simulink model "LLC_bidirectional"  (R2020b)
settings: Solver=ode23tb  StartTime=0.0  StopTime=3.0e-3  RelTol=1e-4  EnableMultiTasking=on
PreLoadFcn:
  | Fs=13000;    % Switching frequency (Hz)
  | Vf=0.6;        % Diode forward voltage (V)
  | Rs_fet=1e5;  % FET snubber resistance (ohms)
  | Cs_fet=1e-5;  % FET snubber capacitance (ohms)
libraries: powerlib x29, powerlib_meascontrol x3, pid_lib x1
Description:
  | Copyright 2008-2019 The MathWorks, Inc.
settings Model: Creator=MathWorks  LastModifiedBy=lauramarks2
settings SolverCC: SolverResetMethod=Robust
settings DataIOCC: SaveOutput=off  SignalLogging=off  DSMLogging=off  SaveTime=off  ReturnWorkspaceOutputs=off
settings OptimizationCC: LifeSpan=inf
settings DebuggingCC: ReadBeforeWriteMsg=DisableAll  WriteAfterWriteMsg=DisableAll  WriteAfterReadMsg=DisableAll  MultiTaskDSMMsg=none  UnconnectedLineMsg=none  SFUnexpectedBacktrackingDiag=warning  SFNoUnconditionalDefaultTransitionDiag=warning  SFExecutionAtInitializationDiag=none  ArithmeticOperatorsInVariantConditions=warning
settings ModelReferenceCC: UpdateModelReferenceTargets=IfOutOfDate
settings SFSimCC: SFSimEcho=off  SimUseLocalCustomCode=off  CustomCodeUndefinedFunction=UseInterfaceOnly
settings RTWCC: RTWUseLocalCustomCode=off
settings CodeAppCC: StateflowObjectComments=on
settings GRTTargetCC: TargetLangStandard=C89/C90 (ANSI)
settings ConfigComp: CovMetricSettings=dw  CovSaveCumulativeToWorkspaceVar=on  CovSaveSingleToWorkspaceVar=on  CovExternalEMLEnable=off
settings SimscapeCC: SimscapeNormalizeSystem=off  SimscapeNominalValues={1, 'bar'; 1, 'cm^3/s'; 1, 'bar*kg/s'; 1, 'kJ/kg'; 1, 'kW'; }

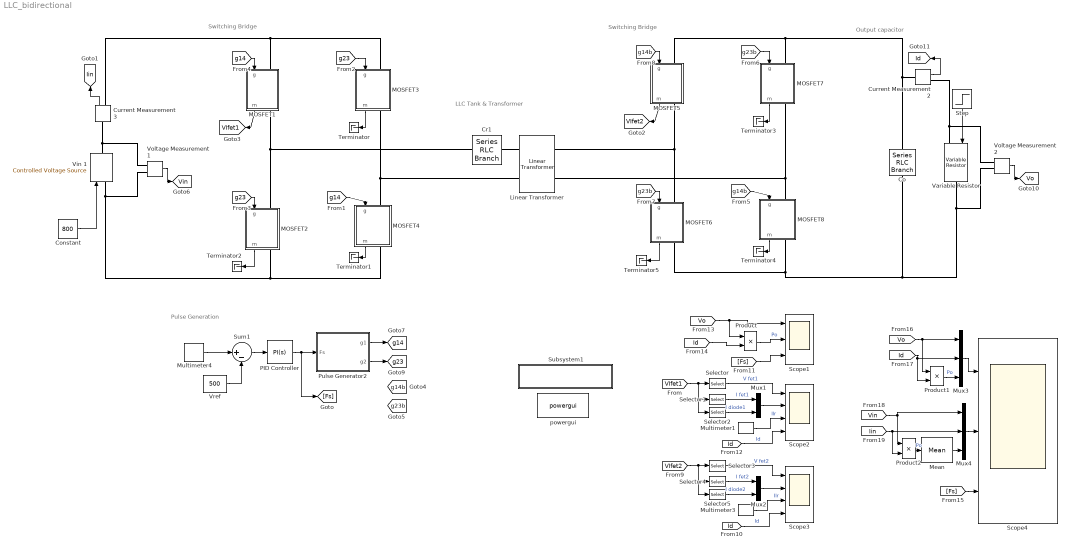
== system LLC_bidirectional ==
  note: Pulse Generation
  note: Switching Bridge
  note: Output capacitor
  note: LLC Tank & Transformer
  note: Switching Bridge
  Co : powerlib/Elements/Series RLC Branch  LConnTagsString=__new0  RConnTagsString=__new0  BranchType=C  Resistance=1e-4  Inductance=200e-6  SetiL0=off  InitialCurrent=0  Capacitance=100e-6  Setx0=on  InitialVoltage=0  Measurements=Branch voltage
  Constant : Constant  Value=800  OutDataTypeStr=double
  Cr1 : powerlib/Elements/Series RLC Branch  LConnTagsString=__new0  RConnTagsString=__new0  BranchType=C  Resistance=1e-4  Inductance=200e-6  SetiL0=off  InitialCurrent=0  Capacitance=1.5e-6  Setx0=off  InitialVoltage=40  Measurements=Branch voltage and current
  Current Measurement2 : powerlib/Measurements/Current Measurement  PhasorSimulation=off  OutputType=Complex  PSBequivalent=0
  Current Measurement3 : powerlib/Measurements/Current Measurement  PhasorSimulation=off  OutputType=Complex  PSBequivalent=0
  Linear Transformer : powerlib/Elements/Linear Transformer  UNITS=SI  NominalPower=[ 100e3 85e3 ]  winding1="[8   1e-2  2.02e-6]"  winding2="[5.7  1e-2  1.16e-6 ]"  ThreeWindings=off  winding3=[3.15e+05 0.7938 0.084225]  RmLm=[1e4 963e-6]  Measurements=All voltages and currents  DataType=on
  MOSFET1 : Subsystem
  MOSFET2 : Subsystem
  MOSFET3 : Subsystem
  MOSFET4 : Subsystem
  MOSFET5 : Subsystem
  MOSFET6 : Subsystem
  MOSFET7 : Subsystem
  MOSFET8 : Subsystem
  Mean : powerlib_meascontrol/Measurements/Mean  Freq=180e3  Vinit=0  Ts=0
  Multimeter1 : powerlib/Measurements/Multimeter  PhasorSimulation=off  OutputType=Complex  sel=1  L=10  Gain=0  yselected={}  PSBOutputType=1  PSBequivalent=0  AxesSetting=[0,0.1,-100,100]  Display=0  SavedBlockNames=-11
  Multimeter3 : powerlib/Measurements/Multimeter  PhasorSimulation=off  OutputType=Complex  sel=1  L=10  Gain=0  yselected={}  PSBOutputType=1  PSBequivalent=0  AxesSetting=[0,0.1,-100,100]  Display=0  SavedBlockNames=-11
  Multimeter4 : powerlib/Measurements/Multimeter  PhasorSimulation=off  OutputType=Complex  sel=1  L=10  Gain=1  yselected={'Ub: Co'};  PSBOutputType=1  PSBequivalent=0  AxesSetting=[0,0.1,-100,100]  Display=0  SavedBlockNames=-11
  Mux1 : Mux  Inputs=2
  Mux2 : Mux  Inputs=2
  Mux3 : Mux  Inputs=3
  Mux4 : Mux  Inputs=3
  PID Controller : pid_lib/PID Controller  Controller=PI  Form=Parallel  TimeDomain=Continuous-time  UseExternalTs=off  SampleTime=-1  IntegratorMethod=Forward Euler  FilterMethod=Forward Euler  ControllerParametersSource=internal  P=1200  I=1e-3  D=0  UseFilter=on  N=100  TunerSelectOption=Transfer Function Based (PID Tuner App)  InitialConditionSource=internal  InitialConditionForIntegrator=89e3  InitialConditionForFilter=0  DifferentiatorICPrevScaledInput=0  ExternalReset=none  TrackingMode=off  Kt=1  LimitOutput=off  SatLimitsSource=internal  UpperSaturationLimit=inf  LowerSaturationLimit=50e3  LinearizeAsGain=off  AntiWindupMode=none  Kb=1  POutMin=[]  POutMax=[]  IOutMin=[]  IOutMax=[]  DOutMin=[]  DOutMax=[]  NOutMin=[]  NOutMax=[]  SumOutMin=[]  SumOutMax=[]  SaturationOutMin=[]  SaturationOutMax=[]  PParamMin=[]  PParamMax=[]  IParamMin=[]  IParamMax=[]  DParamMin=[]  DParamMax=[]  NParamMin=[]  NParamMax=[]  KbParamMin=[]  KbParamMax=[]  KtParamMin=[]  KtParamMax=[]  KbOutMin=[]  KbOutMax=[]  KtOutMin=[]  KtOutMax=[]  IntegratorOutMin=[]  IntegratorOutMax=[]  FilterOutMin=[]  FilterOutMax=[]  SumI1OutMin=[]  SumI1OutMax=[]  SumI2OutMin=[]  SumI2OutMax=[]  SumI3OutMin=[]  SumI3OutMax=[]  SumI4OutMin=[]  SumI4OutMax=[]  SumDOutMin=[]  SumDOutMax=[]  DifferentiatorOutMin=[]  DifferentiatorOutMax=[]  FilterDiffOutCoefMin=[]  FilterDiffOutCoefMax=[]  ReciprocalOutMin=[]  ReciprocalOutMax=[]  SumDenOutMin=[]  SumDenOutMax=[]  SumNumOutMin=[]  SumNumOutMax=[]  DivideOutMin=[]  DivideOutMax=[]  UdiffTsProdOutMin=[]  UdiffTsProdOutMax=[]  NTsProdOutMin=[]  NTsProdOutMax=[]  UintegralTsProdOutMin=[]  UintegralTsProdOutMax=[]  UngainTsProdOutMin=[]  UngainTsProdOutMax=[]  IntegratorContinuousStateAttributes=''  IntegratorStateMustResolveToSignalObject=off  IntegratorRTWStateStorageClass=Auto  FilterContinuousStateAttributes=''  FilterStateMustResolveToSignalObject=off  FilterRTWStateStorageClass=Auto  ParallelPVariant=InternalParameters  IdealPVariant=Disabled  IVariant=InternalParameters  DVariant=Disabled  IntegratorVariant=Continuous  SatVariant=Disabled  AWVariant=Passthrough  PCopyVariant=Disabled  TRVariant=Disabled  FdbkBlocksVariant=Forward  IdealPFdbkVariant=Disabled  SatFdbkVariant=Disabled  DerivativeFilterVariant=Disabled  NVariant=Disabled  NCopyVariant=Disabled_SignalSpec  FilterICVariant=Disabled  IntegratorICVariant=InternalICs  ExternalResetVariant=Disabled  TRSumVariant=Passthrough  SumFdbkVariant=Disabled  SumVariant=Sum_PI  TsampFilterVariant=InternalTs  TsampNgainVariant=Passthrough  TsampIntegralVariant=Passthrough  ExternalSaturationOutDataTypeStr=Inherit: Same as second input
  Product : Product
  Product1 : Product
  Product2 : Product
  Pulse Generator2 : Subsystem
  "Scope1 " : Scope  NumInputPorts=3
  Scope2 : Scope  NumInputPorts=4
  Scope3 : Scope  NumInputPorts=4
  Scope4 : Scope  NumInputPorts=3
  Selector : Selector  InputPortWidth=3  IndexOptions=Index vector (dialog)  Indices=2  OutputSizes=1
  Selector1 : Selector  InputPortWidth=3  IndexOptions=Index vector (dialog)  Indices=1  OutputSizes=1
  Selector2 : Selector  InputPortWidth=3  IndexOptions=Index vector (dialog)  Indices=3  OutputSizes=1
  Selector3 : Selector  InputPortWidth=3  IndexOptions=Index vector (dialog)  Indices=2  OutputSizes=1
  Selector4 : Selector  InputPortWidth=3  IndexOptions=Index vector (dialog)  Indices=1  OutputSizes=1
  Selector5 : Selector  InputPortWidth=3  IndexOptions=Index vector (dialog)  Indices=3  OutputSizes=1
  Step : Step  Time=2e-3  Before=2.5  After=2.5  SampleTime=1e-5
  Subsystem1 : Subsystem
      settings: OpenFcn=|
      | %
      | L=10e-6;
      | C=20e-6;
      | Freq=[1000:1:50000];
      | w=2*pi*Freq;
      | Fo=1/(2*pi*sqrt(L*C));
      | wo=2*pi*Fo;
      | %
      | Rload=[0.5 5];
      | R=8/(pi^2)*Rload;
      | %
      | for n=1:2
      | Q(n)=sqrt(L/C)/R(n);
      |     Zeta(n)=1/(2*Q(n));
      |     s=j*w;
      |     Num(n,:)= (2*Zeta(n)*wo).*s;
      |     Den(n,:)= s.^2 + (2*Zeta(n)*wo).*s + wo^2;
      |     K(n,:)=Num(n,:)./Den(n,:);
      | end
      | figure(1)
      | clf
      | ScreenS=get(0,'Screensize');
      | x0=ScreenS(3); y0=ScreenS(4);
      | PositionParam=[x0/4 y0/8 x0/2 y0/1.4];
      | set(gcf,'Position',PositionParam);
      | subplot(2,1,1)
      | plot(Freq/1000, abs(K(1,:)),'b')
      | hold on
      | plot(Freq/1000, abs(K(2,:)),'r')
      | xlabel('Fs (kHz)')
      | grid
      | axis([0 40 0 1.1])
      | legend('Rload=0.5 ohms', 'Rload=5 ohms','Location', 'NorthEast')
      | title('DC Gain Characteristic - Magnitude')
      | %
      | subplot(2,1,2)
      | plot(Freq/1000, angle(K(1,:))*180/pi,'b')
      | hold on
      | plot(Freq/1000, angle(K(2,:))*180/pi,'r')
      | xlabel('Fs (kHz)')
      | ylabel('Degrees')
      | grid
      | axis([0 40 -100 100])
      | legend('Rload=0.5 ohms', 'Rload=5 ohms','Location', 'NorthEast')
      | title('DC Gain Characteristic - Phase')
      mask Display: disp('Plot Theoretical\nDC Gain Characteristic')
  Sum1 : Sum  Inputs=|+-  InputSameDT=on  SaturateOnIntegerOverflow=on  OutDataTypeStr=Inherit: Same as first input
  Terminator{,1..5} (6 alike) : Terminator
  Variable Resistor : powerlib/Elements/Variable Resistor  Rabsmin=1e-3
      settings: SourceProductBaseCode=PS
  Vin 1 : powerlib/Electrical Sources/Controlled Voltage Source  Initialize=on  Source_Type=AC  Amplitude=0  Phase=0  Frequency=0  Measurements=None
  Voltage Measurement1 : powerlib/Measurements/Voltage Measurement  PhasorSimulation=off  OutputType=Complex  PSBequivalent=0
  Voltage Measurement2 : powerlib/Measurements/Voltage Measurement  PhasorSimulation=off  OutputType=Complex  PSBequivalent=0
  Vref : Constant  Value=500
  powergui : powerlib/powergui  Priority=1  SimulationMode=Discrete  SampleTime=1e-8  frequency=60  Iterations=50  frequencyindice=0  Pbase=100e6  ErrMax=1e-4  UnitsV=kV  UnitsW=MW  buscounter=0  FunctionMessages=off  echomessages=off  EnableUseOfTLC=off  CurrentSourceSwitches=off  DisableSnubberDevices=off  DisableRonSwitches=off  DisableVfSwitches=off  DisplayEquations=off  AutomaticDiscreteSolvers=off  SolverType=Tustin/Backward Euler (TBE)  Interpol=off  ExternalGateDelay=off  methode=off  Ts=100  x0status=blocks  SPID=on  SwTol=0  HookPort=off  NonlinearTolerance=0  nMaxIteration=15  ContinueOnMaxIteration=off  RestoreLinks=warning  ResistiveCurrentMeasurement=off  Frange=[1000:0.5:40000]  Ylog=off  Xlog=off  ShowGrid=off  save=off  variable=ZData  structure=0  ZoomFFT=off  StartTime=0.0  cycles=1  DisplayStyle=1  fundamental=60  FreqAxis=off  MaxFrequency=1000  frequencyindicesteady=1  RmsSteady=1  display=off
  tag scope: Id=global, Iin=global, VIfet1=global, VIfet2=global, Vin=global, Vo=global, g14=global, g14b=global, g23=global, g23b=global
  wires:
  [g23] -> MOSFET2/1(g)
  [g14] -> MOSFET1/1(g)
  MOSFET1/1(m) -> [VIfet1]
  Product/1 -> "Scope1 "/2  "Po"
  [g14] -> MOSFET4/1(g)
  [g23] -> MOSFET3/1(g)
  Mux1/1 -> Scope2/2
  Selector2/1 -> Mux1/2  "I diode1"
  [Id] -> Scope2/4  "Id"
  Multimeter1/1 -> Scope2/3  "Ilr"
  Selector1/1 -> Mux1/1  "I fet1"
  MOSFET3/1(m) -> Terminator/1
  MOSFET4/1(m) -> Terminator1/1
  MOSFET2/1(m) -> Terminator2/1
  [VIfet1] -> Selector2/1, Selector1/1, Selector/1
  Selector/1 -> Scope2/1  "V fet1"
  Current Measurement3/1 -> [Iin]
  Voltage Measurement1/1 -> [Vin]
  MOSFET7/1(m) -> Terminator3/1
  [g23b] -> MOSFET6/1(g)
  [g14b] -> MOSFET8/1(g)
  [g23b] -> MOSFET7/1(g)
  MOSFET5/1(m) -> [VIfet2]
  MOSFET6/1(m) -> Terminator5/1
  [g14b] -> MOSFET5/1(g)
  MOSFET8/1(m) -> Terminator4/1
  Multimeter3/1 -> Scope3/3  "Ilr"
  [Id] -> Scope3/4  "Id"
  Mux2/1 -> Scope3/2
  Selector4/1 -> Mux2/1  "I fet2"
  Selector3/1 -> Scope3/1  "V fet2"
  [VIfet2] -> Selector5/1, Selector4/1, Selector3/1
  Selector5/1 -> Mux2/2  "I diode2"
  Multimeter4/1 -> Sum1/1
  Sum1/1 -> PID Controller/1
  Vref/1 -> Sum1/2
  Pulse Generator2/2(g2) -> [g23]
  Pulse Generator2/1(g1) -> [g14]
  [Fs] -> "Scope1 "/3
  PID Controller/1 -> [Fs], Pulse Generator2/1(Fs)
  Constant/1 -> Vin 1/1
  Step/1 -> Variable Resistor/1
  Voltage Measurement2/1 -> [Vo]
  [Vo] -> Product/1, "Scope1 "/1
  [Id] -> Product/2
  Current Measurement2/1 -> [Id]
  [Vo] -> Product1/1, Mux3/1
  [Id] -> Product1/2, Mux3/2
  Mux3/1 -> Scope4/1
  Product1/1 -> Mux3/3  "Po"
  Mux4/1 -> Scope4/2
  [Vin] -> Product2/1, Mux4/1
  [Iin] -> Product2/2, Mux4/2
  [Fs] -> Scope4/3
  Product2/1 -> Mean/1  "Po"
  Mean/1 -> Mux4/3
  connections:
  MOSFET3/LConn1 -- MOSFET1/LConn1 -- Current Measurement3/RConn1
  Variable Resistor/LConn1 -- Current Measurement2/RConn1 -- Voltage Measurement2/LConn1
  MOSFET3/RConn1 -- Linear Transformer/LConn2 -- MOSFET4/LConn1
  Linear Transformer/LConn1 -- Cr1/RConn1
  MOSFET4/RConn1 -- MOSFET2/RConn1 -- Voltage Measurement1/LConn2 -- Vin 1/LConn1
  Vin 1/RConn1 -- Voltage Measurement1/LConn1 -- Current Measurement3/LConn1
  MOSFET8/RConn1 -- Voltage Measurement2/LConn2 -- Variable Resistor/RConn1 -- Co/RConn1 -- MOSFET6/RConn1
  MOSFET6/LConn1 -- MOSFET5/RConn1 -- Linear Transformer/RConn1
  MOSFET5/LConn1 -- Co/LConn1 -- Current Measurement2/LConn1 -- MOSFET7/LConn1
  MOSFET2/LConn1 -- Cr1/LConn1 -- MOSFET1/RConn1
  MOSFET7/RConn1 -- Linear Transformer/RConn2 -- MOSFET8/LConn1

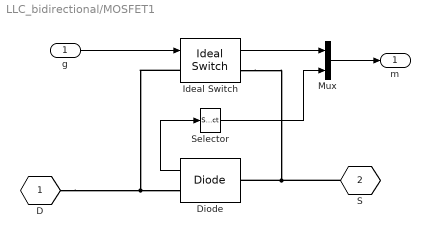
== system LLC_bidirectional/MOSFET1 ==
  g : Inport
  Diode : powerlib/Power Electronics/Diode  Ron=1e-3  Lon=0  Vf=Vf  IC=0  UseSnubber=0  Rs=inf  Cs=0  Measurements=on
  Ideal Switch : powerlib/Power Electronics/Ideal Switch  Ron=1e-3  Lon=0  IC=0  Rs=Rs_fet  Cs=Cs_fet  Measurements=on
  Mux : Mux  Inputs=[2,1]
  Selector : Selector  InputPortWidth=2  IndexOptions=Index vector (dialog)  Indices=1  OutputSizes=1
  D : PMIOPort  Tag=PMCPort  Side=Left
  S : PMIOPort  Tag=PMCPort  Port=2  Side=Right
  m : Outport  VectorParamsAs1DForOutWhenUnconnected=off
  wires:
  Mux/1 -> m/1
  Selector/1 -> Mux/2
  Ideal Switch/1 -> Mux/1
  g/1 -> Ideal Switch/1
  Diode/1 -> Selector/1
  connections:
  Ideal Switch/LConn1 -- D/RConn1 -- Diode/RConn1
  Ideal Switch/RConn1 -- S/RConn1 -- Diode/LConn1

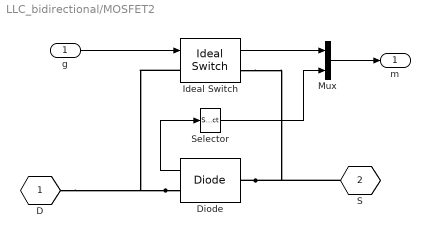
== system LLC_bidirectional/MOSFET2 ==
  g : Inport
  Diode : powerlib/Power Electronics/Diode  Ron=1e-3  Lon=0  Vf=Vf  IC=0  UseSnubber=0  Rs=inf  Cs=0  Measurements=on
  Ideal Switch : powerlib/Power Electronics/Ideal Switch  Ron=1e-3  Lon=0  IC=0  Rs=Rs_fet  Cs=Cs_fet  Measurements=on
  Mux : Mux  Inputs=[2,1]
  Selector : Selector  InputPortWidth=2  IndexOptions=Index vector (dialog)  Indices=1  OutputSizes=1
  D : PMIOPort  Tag=PMCPort  Side=Left
  S : PMIOPort  Tag=PMCPort  Port=2  Side=Right
  m : Outport  VectorParamsAs1DForOutWhenUnconnected=off
  wires:
  Diode/1 -> Selector/1
  g/1 -> Ideal Switch/1
  Ideal Switch/1 -> Mux/1
  Selector/1 -> Mux/2
  Mux/1 -> m/1
  connections:
  Diode/LConn1 -- S/RConn1 -- Ideal Switch/RConn1
  Diode/RConn1 -- D/RConn1 -- Ideal Switch/LConn1

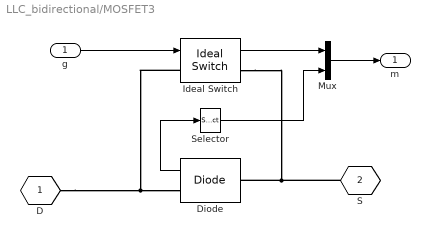
== system LLC_bidirectional/MOSFET3 ==
  g : Inport
  Diode : powerlib/Power Electronics/Diode  Ron=1e-3  Lon=0  Vf=Vf  IC=0  UseSnubber=0  Rs=inf  Cs=0  Measurements=on
  Ideal Switch : powerlib/Power Electronics/Ideal Switch  Ron=1e-3  Lon=0  IC=0  Rs=Rs_fet  Cs=Cs_fet  Measurements=on
  Mux : Mux  Inputs=[2,1]
  Selector : Selector  InputPortWidth=2  IndexOptions=Index vector (dialog)  Indices=1  OutputSizes=1
  D : PMIOPort  Tag=PMCPort  Side=Left
  S : PMIOPort  Tag=PMCPort  Port=2  Side=Right
  m : Outport  VectorParamsAs1DForOutWhenUnconnected=off
  wires:
  Mux/1 -> m/1
  Selector/1 -> Mux/2
  Ideal Switch/1 -> Mux/1
  g/1 -> Ideal Switch/1
  Diode/1 -> Selector/1
  connections:
  Ideal Switch/LConn1 -- D/RConn1 -- Diode/RConn1
  Ideal Switch/RConn1 -- S/RConn1 -- Diode/LConn1

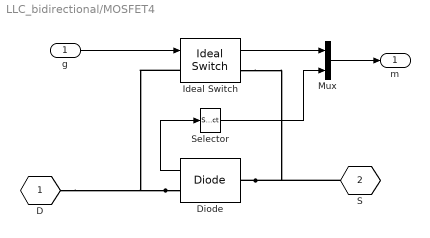
== system LLC_bidirectional/MOSFET4 ==
  g : Inport
  Diode : powerlib/Power Electronics/Diode  Ron=1e-3  Lon=0  Vf=Vf  IC=0  UseSnubber=0  Rs=inf  Cs=0  Measurements=on
  Ideal Switch : powerlib/Power Electronics/Ideal Switch  Ron=1e-3  Lon=0  IC=0  Rs=Rs_fet  Cs=Cs_fet  Measurements=on
  Mux : Mux  Inputs=[2,1]
  Selector : Selector  InputPortWidth=2  IndexOptions=Index vector (dialog)  Indices=1  OutputSizes=1
  D : PMIOPort  Tag=PMCPort  Side=Left
  S : PMIOPort  Tag=PMCPort  Port=2  Side=Right
  m : Outport  VectorParamsAs1DForOutWhenUnconnected=off
  wires:
  Diode/1 -> Selector/1
  g/1 -> Ideal Switch/1
  Ideal Switch/1 -> Mux/1
  Selector/1 -> Mux/2
  Mux/1 -> m/1
  connections:
  Diode/LConn1 -- S/RConn1 -- Ideal Switch/RConn1
  Diode/RConn1 -- D/RConn1 -- Ideal Switch/LConn1

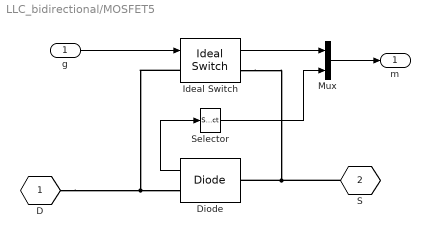
== system LLC_bidirectional/MOSFET5 ==
  g : Inport
  Diode : powerlib/Power Electronics/Diode  Ron=1e-3  Lon=0  Vf=Vf  IC=0  UseSnubber=0  Rs=inf  Cs=0  Measurements=on
  Ideal Switch : powerlib/Power Electronics/Ideal Switch  Ron=1e-3  Lon=0  IC=0  Rs=Rs_fet  Cs=Cs_fet  Measurements=on
  Mux : Mux  Inputs=[2,1]
  Selector : Selector  InputPortWidth=2  IndexOptions=Index vector (dialog)  Indices=1  OutputSizes=1
  D : PMIOPort  Tag=PMCPort  Side=Left
  S : PMIOPort  Tag=PMCPort  Port=2  Side=Right
  m : Outport  VectorParamsAs1DForOutWhenUnconnected=off
  wires:
  Mux/1 -> m/1
  Selector/1 -> Mux/2
  Ideal Switch/1 -> Mux/1
  g/1 -> Ideal Switch/1
  Diode/1 -> Selector/1
  connections:
  Ideal Switch/LConn1 -- D/RConn1 -- Diode/RConn1
  Ideal Switch/RConn1 -- S/RConn1 -- Diode/LConn1

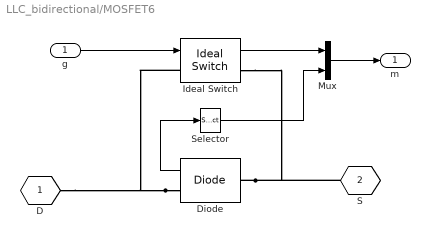
== system LLC_bidirectional/MOSFET6 ==
  g : Inport
  Diode : powerlib/Power Electronics/Diode  Ron=1e-3  Lon=0  Vf=Vf  IC=0  UseSnubber=0  Rs=inf  Cs=0  Measurements=on
  Ideal Switch : powerlib/Power Electronics/Ideal Switch  Ron=1e-3  Lon=0  IC=0  Rs=Rs_fet  Cs=Cs_fet  Measurements=on
  Mux : Mux  Inputs=[2,1]
  Selector : Selector  InputPortWidth=2  IndexOptions=Index vector (dialog)  Indices=1  OutputSizes=1
  D : PMIOPort  Tag=PMCPort  Side=Left
  S : PMIOPort  Tag=PMCPort  Port=2  Side=Right
  m : Outport  VectorParamsAs1DForOutWhenUnconnected=off
  wires:
  Diode/1 -> Selector/1
  g/1 -> Ideal Switch/1
  Ideal Switch/1 -> Mux/1
  Selector/1 -> Mux/2
  Mux/1 -> m/1
  connections:
  Diode/LConn1 -- S/RConn1 -- Ideal Switch/RConn1
  Diode/RConn1 -- D/RConn1 -- Ideal Switch/LConn1

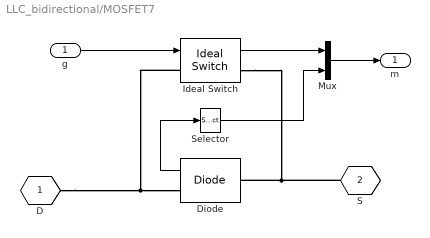
== system LLC_bidirectional/MOSFET7 ==
  g : Inport
  Diode : powerlib/Power Electronics/Diode  Ron=1e-3  Lon=0  Vf=Vf  IC=0  UseSnubber=0  Rs=inf  Cs=0  Measurements=on
  Ideal Switch : powerlib/Power Electronics/Ideal Switch  Ron=1e-3  Lon=0  IC=0  Rs=Rs_fet  Cs=Cs_fet  Measurements=on
  Mux : Mux  Inputs=[2,1]
  Selector : Selector  InputPortWidth=2  IndexOptions=Index vector (dialog)  Indices=1  OutputSizes=1
  D : PMIOPort  Tag=PMCPort  Side=Left
  S : PMIOPort  Tag=PMCPort  Port=2  Side=Right
  m : Outport  VectorParamsAs1DForOutWhenUnconnected=off
  wires:
  Mux/1 -> m/1
  Selector/1 -> Mux/2
  Ideal Switch/1 -> Mux/1
  g/1 -> Ideal Switch/1
  Diode/1 -> Selector/1
  connections:
  Ideal Switch/LConn1 -- D/RConn1 -- Diode/RConn1
  Ideal Switch/RConn1 -- S/RConn1 -- Diode/LConn1

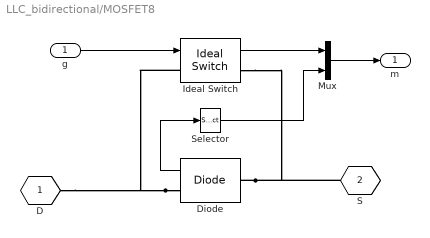
== system LLC_bidirectional/MOSFET8 ==
  g : Inport
  Diode : powerlib/Power Electronics/Diode  Ron=1e-3  Lon=0  Vf=Vf  IC=0  UseSnubber=0  Rs=inf  Cs=0  Measurements=on
  Ideal Switch : powerlib/Power Electronics/Ideal Switch  Ron=1e-3  Lon=0  IC=0  Rs=Rs_fet  Cs=Cs_fet  Measurements=on
  Mux : Mux  Inputs=[2,1]
  Selector : Selector  InputPortWidth=2  IndexOptions=Index vector (dialog)  Indices=1  OutputSizes=1
  D : PMIOPort  Tag=PMCPort  Side=Left
  S : PMIOPort  Tag=PMCPort  Port=2  Side=Right
  m : Outport  VectorParamsAs1DForOutWhenUnconnected=off
  wires:
  Diode/1 -> Selector/1
  g/1 -> Ideal Switch/1
  Ideal Switch/1 -> Mux/1
  Selector/1 -> Mux/2
  Mux/1 -> m/1
  connections:
  Diode/LConn1 -- S/RConn1 -- Ideal Switch/RConn1
  Diode/RConn1 -- D/RConn1 -- Ideal Switch/LConn1

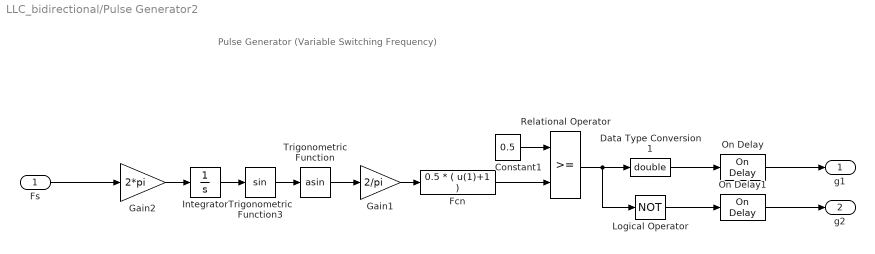
== system LLC_bidirectional/Pulse Generator2 ==
  note: Pulse Generator
      | (Variable Switching Frequency)
  Fs : Inport
  Constant1 : Constant  Value=0.5
  Data Type Conversion1 : DataTypeConversion  OutDataTypeStr=double
  Fcn : Fcn  Expr=0.5 * ( u(1)+1 )
  Gain1 : Gain  Gain=2/pi  SaturateOnIntegerOverflow=on  OutDataTypeStr=Inherit: Same as input  ParamDataTypeStr=Inherit: Same as input
  Gain2 : Gain  Gain=2*pi  SaturateOnIntegerOverflow=on  OutDataTypeStr=Inherit: Same as input  ParamDataTypeStr=Inherit: Same as input
  Integrator : Integrator
  Logical Operator : Logic  Operator=NOT  AllPortsSameDT=off  OutDataTypeStr=float('double')
  On Delay : powerlib_meascontrol/Logic/On Delay  DelayType=On delay  delay=400e-9  ic=0  Ts=0
  On Delay1 : powerlib_meascontrol/Logic/On Delay  DelayType=On delay  delay=400e-9  ic=0  Ts=0
  Relational Operator : RelationalOperator  OutDataTypeStr=boolean  RndMeth=Nearest
  Trigonometric Function : Trigonometry  Operator=asin
  Trigonometric Function3 : Trigonometry
  g1 : Outport  VectorParamsAs1DForOutWhenUnconnected=off
  g2 : Outport  Port=2  VectorParamsAs1DForOutWhenUnconnected=off
  wires:
  On Delay1/1 -> g2/1
  On Delay/1 -> g1/1
  Fs/1 -> Gain2/1
  Gain2/1 -> Integrator/1
  Data Type Conversion1/1 -> On Delay/1
  Logical Operator/1 -> On Delay1/1
  Fcn/1 -> Relational Operator/2
  Relational Operator/1 -> Logical Operator/1, Data Type Conversion1/1
  Constant1/1 -> Relational Operator/1
  Integrator/1 -> Trigonometric Function3/1
  Trigonometric Function/1 -> Gain1/1
  Gain1/1 -> Fcn/1
  Trigonometric Function3/1 -> Trigonometric Function/1

== system LLC_bidirectional/Subsystem1 ==
